simulink model "FuelSystemb"  (R2019b)
settings: Solver=FixedStepDiscrete  StartTime=0.0  StopTime=inf  FixedStep=FspSamplingPeriod  RelTol=1e-3
undefined symbols (not defined in the file or in its folder): BooleanOn, Left, OrifaceC, Right
libraries: FuelSystemLibrary x24
settings Model: Creator=sj3-wright  LastModifiedBy=George
settings DataIOCC: LimitDataPoints=on  SaveFormat=Array  ReturnWorkspaceOutputs=off
settings OptimizationCC: BlockReduction=off  BooleanDataType=off  LifeSpan=inf
settings DebuggingCC: SaveWithParameterizedLinksMsg=none  UnderspecifiedInitializationDetection=Classic  MergeDetectMultiDrivingBlocksExec=none  SignalResolutionControl=TryResolveAllWithWarning  SFUnexpectedBacktrackingDiag=warning  SFNoUnconditionalDefaultTransitionDiag=warning  SFExecutionAtInitializationDiag=none  ArithmeticOperatorsInVariantConditions=warning
settings HardwareCC: ProdBitPerPointer=32  ProdBitPerSizeT=32  ProdBitPerPtrDiffT=32  ProdLargestAtomicFloat=None  ProdIntDivRoundTo=Undefined  ProdEndianess=Unspecified  ProdWordSize=32  ProdHWDeviceType=32-bit Generic  TargetUnknown=on
settings ModelReferenceCC: PropagateSignalLabelsOutOfModel=off
settings SFSimCC: SimUseLocalCustomCode=off  CustomCodeUndefinedFunction=UseInterfaceOnly
settings RTWCC: RTWUseLocalCustomCode=off
settings CodeAppCC: StateflowObjectComments=on
settings GRTTargetCC: TargetLangStandard=C89/C90 (ANSI)
settings ConfigComp: CovMetricSettings=dw  CovSaveCumulativeToWorkspaceVar=on  CovSaveSingleToWorkspaceVar=on  CovExternalEMLEnable=off  CovSFcnEnable=off

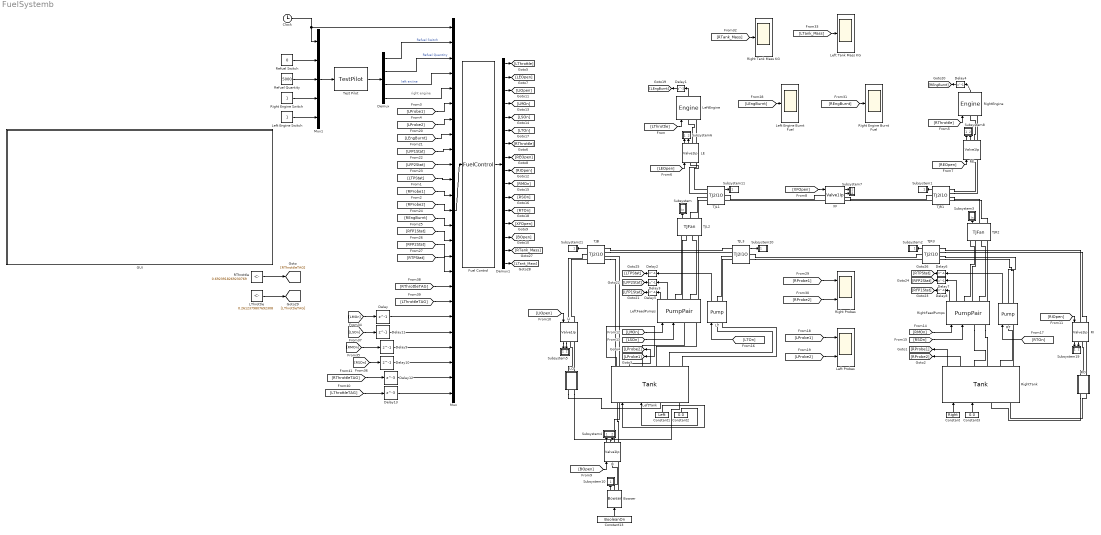
== system FuelSystemb ==
  note: right engine
  B : FuelSystemLibrary/Valve1Ip  SystemSampleTime=-1  Latency=0  AutoFrameSizeCalculation=off
  Bowser : FuelSystemLibrary/Bowser  SystemSampleTime=-1  Latency=0  AutoFrameSizeCalculation=off
  Clock : Clock
  Constant : Constant  Value=Right
  Constant1 : Constant  Value=Left
  Constant13 : Constant  Value=BooleanOn
  Constant2 : Constant  Value=0.0
  Constant3 : Constant  Value=0.0
  Delay{,1..11} (12 alike) : Delay  DelayLength=1  InitialCondition=0
  Delay12 : Delay  DelayLength=3  InitialCondition=0
  Delay13 : Delay  DelayLength=3  InitialCondition=0
  Demux : Demux
  Demux1 : Demux  Outputs=16
  Fuel Control : MATLABFcn  MATLABFcn=FuelControl  OutputDimensions=[16]
  GUI : Subsystem
  LE : FuelSystemLibrary/Valve1Ip  SystemSampleTime=-1  Latency=0  AutoFrameSizeCalculation=off
  LI : FuelSystemLibrary/Valve1Ip  SystemSampleTime=-1  Latency=0  AutoFrameSizeCalculation=off
  LO : Subsystem
  LT : FuelSystemLibrary/Pump  SystemSampleTime=-1  Latency=0  AutoFrameSizeCalculation=off
  LThrottle : Constant  Value=0.2612379807692308
  Left Engine Burnt Fuel : Scope
  Left Engine Switch : Constant
  Left Probes : Scope  NumInputPorts=2
  Left Tank Mass KG : Scope
  LeftEngine : FuelSystemLibrary/Engine  SystemSampleTime=-1  Latency=0  AutoFrameSizeCalculation=off
      link override Constant10: Value=0
  LeftFeedPumps : FuelSystemLibrary/PumpPair  SystemSampleTime=-1  Latency=0  AutoFrameSizeCalculation=off
  LeftTank : FuelSystemLibrary/Tank  SystemSampleTime=-1  Latency=0  AutoFrameSizeCalculation=off
  Mux : Mux  Inputs=25
  Mux1 : Mux  Inputs=5
  RE : FuelSystemLibrary/Valve1Ip  SystemSampleTime=-1  Latency=0  AutoFrameSizeCalculation=off
  RI : FuelSystemLibrary/Valve1Ip  SystemSampleTime=-1  Latency=0  AutoFrameSizeCalculation=off
  RO : Subsystem
  RT : FuelSystemLibrary/Pump  SystemSampleTime=-1  Latency=0  AutoFrameSizeCalculation=off
  RThrottle : Constant  Value=0.6923918269230769
  Refuel Quantity : Constant  Value=5000
  Refuel Switch : Constant  Value=0
  Right Engine Burnt Fuel : Scope
  Right Engine Switch : Constant
  Right Probes : Scope  NumInputPorts=2
  Right Tank Mass KG : Scope
  RightEngine : FuelSystemLibrary/Engine  SystemSampleTime=-1  Latency=0  AutoFrameSizeCalculation=off
  RightFeedPumps : FuelSystemLibrary/PumpPair  SystemSampleTime=-1  Latency=0  AutoFrameSizeCalculation=off
  RightTank : FuelSystemLibrary/Tank  SystemSampleTime=-1  Latency=0  AutoFrameSizeCalculation=off
  Subsystem : Subsystem
  Subsystem1 : Subsystem
  Subsystem10 : Subsystem
  Subsystem11 : Subsystem
  Subsystem19 : Subsystem
  Subsystem2 : Subsystem
  Subsystem20 : Subsystem
  Subsystem21 : Subsystem
  Subsystem3 : Subsystem
  Subsystem4 : Subsystem
  Subsystem5 : Subsystem
  Subsystem6 : Subsystem
  Subsystem7 : Subsystem
  Subsystem8 : Subsystem
  TJB : FuelSystemLibrary/TJ2I1O  SystemSampleTime=-1  Latency=0  AutoFrameSizeCalculation=off
  TJL1 : FuelSystemLibrary/TJ2I1O  SystemSampleTime=-1  Latency=0  AutoFrameSizeCalculation=off
  TJL2 : FuelSystemLibrary/TJFan  SystemSampleTime=-1  Latency=0  AutoFrameSizeCalculation=off
  TJL3 : FuelSystemLibrary/TJ2I1O  SystemSampleTime=-1  Latency=0  AutoFrameSizeCalculation=off
  TJR1 : FuelSystemLibrary/TJ2I1O  SystemSampleTime=-1  Latency=0  AutoFrameSizeCalculation=off
  TJR2 : FuelSystemLibrary/TJFan  SystemSampleTime=-1  Latency=0  AutoFrameSizeCalculation=off
  TJR3 : FuelSystemLibrary/TJ2I1O  SystemSampleTime=-1  Latency=0  AutoFrameSizeCalculation=off
  Test Pilot : MATLABFcn  MATLABFcn=TestPilot
  XF : FuelSystemLibrary/Valve1Ip  SystemSampleTime=-1  Latency=0  AutoFrameSizeCalculation=off
  wires:
  Constant/1 -> RightTank/1
  Constant1/1 -> LeftTank/1
  Constant2/1 -> LeftTank/2
  Constant3/1 -> RightTank/2
  [RIOpen] -> RI/1
  [BOpen] -> B/1
  [LIOpen] -> LI/1
  [LEOpen] -> LE/1
  [REOpen] -> RE/1
  [RThrottle] -> RightEngine/1
  [LThrottle] -> LeftEngine/1
  [XFOpen] -> XF/1
  Constant13/1 -> Bowser/1
  [LTOn] -> LT/1
  [RTOn] -> RT/1
  RightTank/1 -> [RProbe1]
  RightTank/2 -> [RProbe2]
  LeftTank/1 -> [LProbe1]
  LeftTank/2 -> [LProbe2]
  Clock/1 -> Mux/1, Mux1/1
  [LMOn] -> LeftFeedPumps/1
  [LSOn] -> LeftFeedPumps/2
  [RMOn] -> RightFeedPumps/1
  [RSOn] -> RightFeedPumps/2
  Demux1/11 -> [RSOn]
  Demux1/5 -> [LSOn]
  Demux1/10 -> [RMOn]
  Demux1/12 -> [RTOn]
  Demux1/6 -> [LTOn]
  Demux1/13 -> [XFOpen]
  Demux1/8 -> [REOpen]
  Demux1/7 -> [RThrottle]
  Demux1/9 -> [RIOpen]
  Demux1/14 -> [BOpen]
  Demux1/3 -> [LIOpen]
  Demux1/1 -> [LThrottle]
  Demux1/2 -> [LEOpen]
  Demux1/4 -> [LMOn]
  TJL2/1 -> Subsystem/1(In)
  TJR1/1 -> Subsystem1/1(In)
  TJR3/1 -> Subsystem2/1(In)
  TJR2/1 -> Subsystem3/1(In)
  B/1 -> Subsystem4/1(1)
  B/2 -> Subsystem4/2(2)
  LI/1 -> Subsystem5/1(1)
  LI/2 -> Subsystem5/2(2)
  LE/1 -> Subsystem6/1(1)
  LE/2 -> Subsystem6/2(2)
  XF/1 -> Subsystem7/1(1)
  XF/2 -> Subsystem7/2(2)
  RE/1 -> Subsystem8/1(1)
  RE/2 -> Subsystem8/2(2)
  Bowser/1 -> Subsystem10/1(1)
  TJL1/1 -> Subsystem11/1(In)
  LeftEngine/1 -> Delay1/1
  RightEngine/1 -> Delay4/1
  LT/1 -> Delay2/1
  RightFeedPumps/1 -> Delay8/1
  RightFeedPumps/2 -> Delay7/1
  RT/1 -> Delay6/1
  RI/1 -> Subsystem19/1(1)
  RI/2 -> Subsystem19/2(2)
  TJL3/1 -> Subsystem20/1(In)
  [LProbe1] -> Left Probes/1
  TJB/1 -> Subsystem21/1(In)
  [LProbe2] -> Left Probes/2
  Demux/1 -> Mux/2  "Refuel Switch"
  Demux/2 -> Mux/3  "Refuel Quantity"
  Demux/3 -> Mux/4  "left eniine"
  Test Pilot/1 -> Demux/1
  Mux/1 -> Fuel Control/1
  LeftFeedPumps/1 -> Delay5/1
  LeftFeedPumps/2 -> Delay3/1
  [LProbe2] -> Mux/7
  [LProbe1] -> Mux/6
  [RProbe1] -> Mux/12
  [RProbe2] -> Mux/13
  [REngBurnt] -> Mux/14
  [LFP1Stat] -> Mux/9
  [LFP2Stat] -> Mux/10
  [LTPStat] -> Mux/11
  [RFP1Stat] -> Mux/15
  [RFP2Stat] -> Mux/16
  [RTPStat] -> Mux/17
  Fuel Control/1 -> Demux1/1
  [LEngBurnt] -> Mux/8
  Delay1/1 -> [LEngBurnt]
  Delay4/1 -> [REngBurnt]
  Delay2/1 -> [LTPStat]
  Delay3/1 -> [LFP2Stat]
  Delay5/1 -> [LFP1Stat]
  Delay6/1 -> [RTPStat]
  Delay7/1 -> [RFP2Stat]
  Delay8/1 -> [RFP1Stat]
  [LEngBurnt] -> Left Engine Burnt Fuel/1
  [RProbe1] -> Right Probes/1
  [RProbe2] -> Right Probes/2
  Demux1/16 -> [LTank_Mass]
  Demux1/15 -> [RTank_Mass]
  [RTank_Mass] -> Right Tank Mass KG/1
  [LTank_Mass] -> Left Tank Mass KG/1
  Refuel Switch/1 -> Mux1/2
  Mux1/1 -> Test Pilot/1
  Refuel Quantity/1 -> Mux1/3
  Right Engine Switch/1 -> Mux1/4
  Left Engine Switch/1 -> Mux1/5
  Demux/4 -> Mux/5
  [REngBurnt] -> Right Engine Burnt Fuel/1
  [LMOn] -> Delay/1
  Delay/1 -> Mux/20
  Delay9/1 -> Mux/22
  [RMOn] -> Delay9/1
  Delay10/1 -> Mux/23
  [RSOn] -> Delay10/1
  Delay11/1 -> Mux/21
  [LSOn] -> Delay11/1
  Delay12/1 -> Mux/24
  Delay13/1 -> Mux/25
  RThrottle/1 -> [RThrottleTAG]
  [RThrottleTAG] -> Mux/18
  LThrottle/1 -> [LThrottleTAG]
  [LThrottleTAG] -> Mux/19
  [RThrottleTAG] -> Delay12/1
  [LThrottleTAG] -> Delay13/1
  connections:
  LeftFeedPumps/RConn1 -- TJL2/LConn1
  LeftFeedPumps/RConn2 -- TJL2/LConn2
  LeftFeedPumps/RConn3 -- TJL2/LConn3
  LeftFeedPumps/RConn4 -- TJL2/LConn4
  LeftTank/RConn1 -- LeftFeedPumps/LConn1
  LeftTank/RConn2 -- LeftFeedPumps/LConn2
  TJL2/RConn2 -- TJL1/LConn4
  TJL2/RConn1 -- TJL1/LConn3
  TJL1/RConn1 -- XF/LConn1
  XF/LConn2 -- TJL1/RConn2
  TJL1/LConn1 -- LE/LConn1
  TJL1/LConn2 -- LE/LConn2
  LE/RConn1 -- LeftEngine/LConn1
  LE/RConn2 -- LeftEngine/LConn2
  LeftTank/RConn4 -- LT/LConn2
  LeftTank/RConn3 -- LT/LConn1
  LT/RConn2 -- TJL3/LConn4
  LT/RConn1 -- TJL3/LConn3
  TJL3/RConn1 -- TJR3/RConn1
  TJL3/RConn2 -- TJR3/RConn2
  TJB/LConn1 -- TJL3/LConn1
  TJB/LConn2 -- TJL3/LConn2
  LI/LConn1 -- TJB/RConn1
  LI/LConn2 -- TJB/RConn2
  Bowser/RConn2 -- B/LConn2
  Bowser/RConn1 -- B/LConn1
  RightFeedPumps/LConn2 -- RightTank/RConn2
  RightFeedPumps/LConn1 -- RightTank/RConn1
  RightTank/RConn4 -- RT/LConn2
  RightTank/RConn3 -- RT/LConn1
  TJR3/LConn3 -- RT/RConn1
  TJR3/LConn4 -- RT/RConn2
  TJR1/LConn4 -- TJR2/RConn2
  TJR1/LConn3 -- TJR2/RConn1
  RE/RConn1 -- RightEngine/LConn1
  RE/RConn2 -- RightEngine/LConn2
  TJR1/LConn1 -- RE/LConn1
  TJR1/LConn2 -- RE/LConn2
  XF/RConn2 -- TJR1/RConn2
  XF/RConn1 -- TJR1/RConn1
  B/RConn1 -- TJB/LConn3
  TJB/LConn4 -- B/RConn2
  TJR3/LConn1 -- RI/LConn1
  TJR3/LConn2 -- RI/LConn2
  LO/LConn2 -- LI/RConn2
  LO/LConn1 -- LI/RConn1
  LO/RConn2 -- LeftTank/LConn2
  LO/RConn1 -- LeftTank/LConn1
  RO/LConn2 -- RI/RConn2
  RO/LConn1 -- RI/RConn1
  RO/RConn2 -- RightTank/LConn2
  RO/RConn1 -- RightTank/LConn1
  RightFeedPumps/RConn4 -- TJR2/LConn4
  RightFeedPumps/RConn3 -- TJR2/LConn3
  RightFeedPumps/RConn2 -- TJR2/LConn2
  RightFeedPumps/RConn1 -- TJR2/LConn1

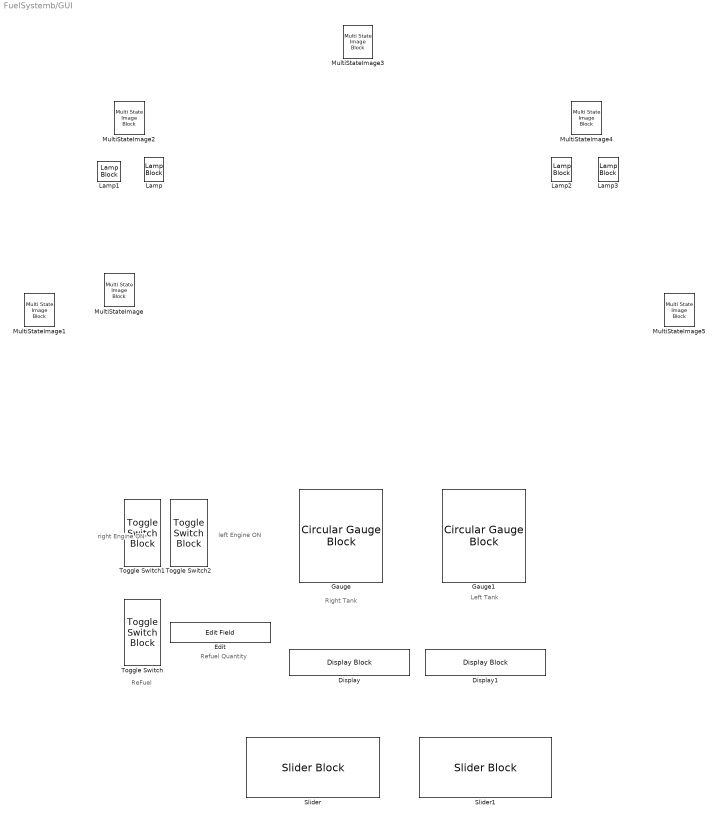
== system FuelSystemb/GUI ==
  note: ReFuel
  note: left Engine ON
  note: Refuel Quantity
  note: right
      | Engine ON
  note: Left Tank
  note: Right Tank
  Display : DisplayBlock  LabelPosition=Hide  Format=shortG  Transparency=1
  Display1 : DisplayBlock  LabelPosition=Hide  Format=shortG  Transparency=1
  Edit : EditField  LabelPosition=Hide  ShowInitialText=on  Alignment=Center
  Gauge : CircularGaugeBlock  LabelPosition=Hide  ScaleMax=3000
  Gauge1 : CircularGaugeBlock  LabelPosition=Hide  ScaleMax=3000
  Lamp{,1..3} (4 alike) : LampBlock  LabelPosition=Hide
  MultiStateImage{,1..5} (6 alike) : MultiStateImageBlock  LabelPosition=Hide
  Slider : SliderBlock  ScaleMin=0.05  ScaleMax=1
  Slider1 : SliderBlock  ScaleMin=0.05  ScaleMax=1
  Toggle Switch : ToggleSwitchBlock  LabelPosition=Hide
      settings: Values={{'Off', 'On'}, [0 1]}
  Toggle Switch1 : ToggleSwitchBlock  LabelPosition=Hide
      settings: Values={{'Off', 'On'}, [0 1]}
  Toggle Switch2 : ToggleSwitchBlock  LabelPosition=Hide
      settings: Values={{'Off', 'On'}, [0 1]}

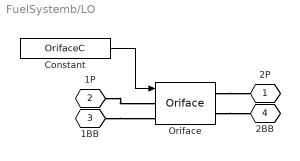
== system FuelSystemb/LO ==
  Constant : Constant  Value=OrifaceC
  Oriface : FuelSystemLibrary/Oriface  SystemSampleTime=-1  Latency=0  AutoFrameSizeCalculation=off
  2P : PMIOPort  Tag=PMCPort  Side=Left
  1P : PMIOPort  Tag=PMCPort  Port=2  Side=Right
  1BB : PMIOPort  Tag=PMCPort  Port=3  Side=Left
  2BB : PMIOPort  Tag=PMCPort  Port=4  Side=Right
  wires:
  Constant/1 -> Oriface/1
  connections:
  1BB/RConn1 -- Oriface/LConn2
  1P/RConn1 -- Oriface/LConn1
  Oriface/RConn2 -- 2BB/RConn1
  Oriface/RConn1 -- 2P/RConn1

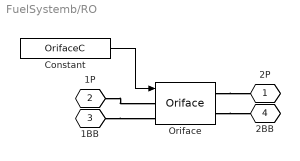
== system FuelSystemb/RO ==
  Constant : Constant  Value=OrifaceC
  Oriface : FuelSystemLibrary/Oriface  SystemSampleTime=-1  Latency=0  AutoFrameSizeCalculation=off
  2P : PMIOPort  Tag=PMCPort  Side=Left
  1P : PMIOPort  Tag=PMCPort  Port=2  Side=Right
  1BB : PMIOPort  Tag=PMCPort  Port=3  Side=Left
  2BB : PMIOPort  Tag=PMCPort  Port=4  Side=Right
  wires:
  Constant/1 -> Oriface/1
  connections:
  1BB/RConn1 -- Oriface/LConn2
  1P/RConn1 -- Oriface/LConn1
  Oriface/RConn2 -- 2BB/RConn1
  Oriface/RConn1 -- 2P/RConn1

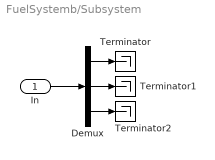
== system FuelSystemb/Subsystem ==
  In : Inport
  Demux : Demux  Outputs=3
  Terminator : Terminator
  Terminator1 : Terminator
  Terminator2 : Terminator
  wires:
  In/1 -> Demux/1
  Demux/1 -> Terminator/1
  Demux/2 -> Terminator1/1
  Demux/3 -> Terminator2/1

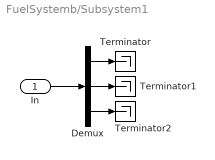
== system FuelSystemb/Subsystem1 ==
  In : Inport
  Demux : Demux  Outputs=3
  Terminator : Terminator
  Terminator1 : Terminator
  Terminator2 : Terminator
  wires:
  In/1 -> Demux/1
  Demux/1 -> Terminator/1
  Demux/2 -> Terminator1/1
  Demux/3 -> Terminator2/1

== system FuelSystemb/Subsystem10 ==
  1 : Inport
  Terminator : Terminator
  wires:
  1/1 -> Terminator/1

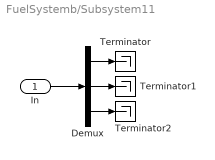
== system FuelSystemb/Subsystem11 ==
  In : Inport
  Demux : Demux  Outputs=3
  Terminator : Terminator
  Terminator1 : Terminator
  Terminator2 : Terminator
  wires:
  In/1 -> Demux/1
  Demux/1 -> Terminator/1
  Demux/2 -> Terminator1/1
  Demux/3 -> Terminator2/1

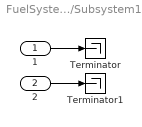
== system FuelSystemb/Subsystem19 ==
  1 : Inport
  2 : Inport  Port=2
  Terminator : Terminator
  Terminator1 : Terminator
  wires:
  1/1 -> Terminator/1
  2/1 -> Terminator1/1

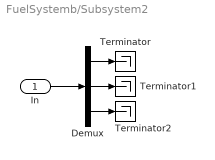
== system FuelSystemb/Subsystem2 ==
  In : Inport
  Demux : Demux  Outputs=3
  Terminator : Terminator
  Terminator1 : Terminator
  Terminator2 : Terminator
  wires:
  In/1 -> Demux/1
  Demux/1 -> Terminator/1
  Demux/2 -> Terminator1/1
  Demux/3 -> Terminator2/1

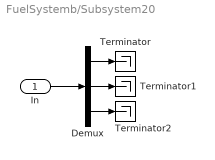
== system FuelSystemb/Subsystem20 ==
  In : Inport
  Demux : Demux  Outputs=3
  Terminator : Terminator
  Terminator1 : Terminator
  Terminator2 : Terminator
  wires:
  In/1 -> Demux/1
  Demux/1 -> Terminator/1
  Demux/2 -> Terminator1/1
  Demux/3 -> Terminator2/1

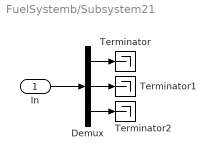
== system FuelSystemb/Subsystem21 ==
  In : Inport
  Demux : Demux  Outputs=3
  Terminator : Terminator
  Terminator1 : Terminator
  Terminator2 : Terminator
  wires:
  In/1 -> Demux/1
  Demux/1 -> Terminator/1
  Demux/2 -> Terminator1/1
  Demux/3 -> Terminator2/1

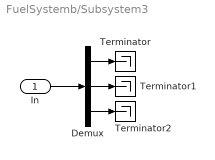
== system FuelSystemb/Subsystem3 ==
  In : Inport
  Demux : Demux  Outputs=3
  Terminator : Terminator
  Terminator1 : Terminator
  Terminator2 : Terminator
  wires:
  In/1 -> Demux/1
  Demux/1 -> Terminator/1
  Demux/2 -> Terminator1/1
  Demux/3 -> Terminator2/1

== system FuelSystemb/Subsystem4 ==
  1 : Inport
  2 : Inport  Port=2
  Terminator : Terminator
  Terminator1 : Terminator
  wires:
  1/1 -> Terminator/1
  2/1 -> Terminator1/1

== system FuelSystemb/Subsystem5 ==
  1 : Inport
  2 : Inport  Port=2
  Terminator : Terminator
  Terminator1 : Terminator
  wires:
  1/1 -> Terminator/1
  2/1 -> Terminator1/1

== system FuelSystemb/Subsystem6 ==
  1 : Inport
  2 : Inport  Port=2
  Terminator : Terminator
  Terminator1 : Terminator
  wires:
  1/1 -> Terminator/1
  2/1 -> Terminator1/1

== system FuelSystemb/Subsystem7 ==
  1 : Inport
  2 : Inport  Port=2
  Terminator : Terminator
  Terminator1 : Terminator
  wires:
  1/1 -> Terminator/1
  2/1 -> Terminator1/1

== system FuelSystemb/Subsystem8 ==
  1 : Inport
  2 : Inport  Port=2
  Terminator : Terminator
  Terminator1 : Terminator
  wires:
  1/1 -> Terminator/1
  2/1 -> Terminator1/1
